simulink model "Headlight_dimmer"  (R2016a)
settings: Solver=VariableStepAuto  StartTime=0.0  StopTime=10.0  RelTol=1e-3
model workspace (MAT data in the model file):
  en = 0
  val = 0
  val1 = 0
values from neighbouring files (symbols this model uses):
  A = 1    [R_calculation_variables.mat]
  a = 0.7    [R_calculation_variables.mat]
libraries: simulink x3
settings Model: Creator=Admin  LastModifiedBy=Admin
settings DataIOCC: ExternalInput=[t, E]

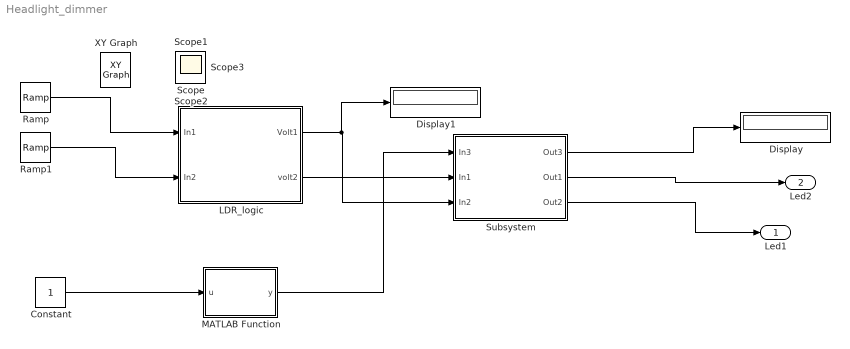
== system Headlight_dimmer ==
  Constant : Constant
  Display : Display
  Display1 : Display
  "LDR_logic " : Subsystem
  MATLAB Function : MATLAB Function  TreatAsAtomicUnit=on
  Ramp : simulink/Sources/Ramp  slope=0.5  start=0  X0=0
  Ramp1 : simulink/Sources/Ramp  slope=0.5  start=0  X0=0
  Subsystem : Subsystem
  Led1 : Outport
  Led2 : Outport  Port=2
  Scope{,1..3} (4 alike) : Scope
  XY Graph : simulink/Sinks/XY Graph  IOType=viewer  xmin=-1  xmax=1  ymin=-1  ymax=1  st=-1
  wires:
  Constant/1 -> MATLAB Function/1(u)
  Ramp/1 -> "LDR_logic "/1(In1)
  Ramp1/1 -> "LDR_logic "/2(In2)
  MATLAB Function/1(y) -> Subsystem/1(In3)
  "LDR_logic "/1(Volt1) -> Display1/1, Subsystem/3(In2)
  "LDR_logic "/2(volt2) -> Subsystem/2(In1)
  Subsystem/1(Out3) -> Display/1
  Subsystem/2(Out1) -> Led2/1
  Subsystem/3(Out2) -> Led1/1

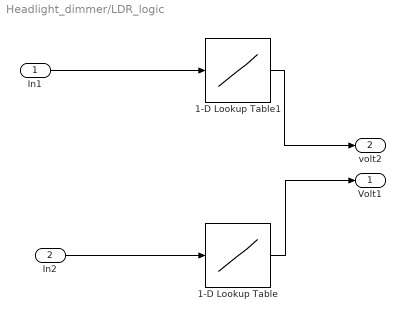
== system Headlight_dimmer/LDR_logic  ==
  In1 : Inport
  In2 : Inport  Port=2
  1-D Lookup Table : Lookup_n-D  NumberOfTableDimensions=1  BreakpointsForDimension1=A.*E.^a  Table=A.*E.^a  InternalRulePriority=Speed  RndMeth=Simplest  InputSameDT=on
  1-D Lookup Table1 : Lookup_n-D  NumberOfTableDimensions=1  BreakpointsForDimension1=A.*E.^a  Table=A.*E.^a  InternalRulePriority=Speed  RndMeth=Simplest  InputSameDT=on
  Volt1 : Outport
  volt2 : Outport  Port=2
  wires:
  1-D Lookup Table1/1 -> volt2/1
  1-D Lookup Table/1 -> Volt1/1
  In1/1 -> 1-D Lookup Table1/1
  In2/1 -> 1-D Lookup Table/1

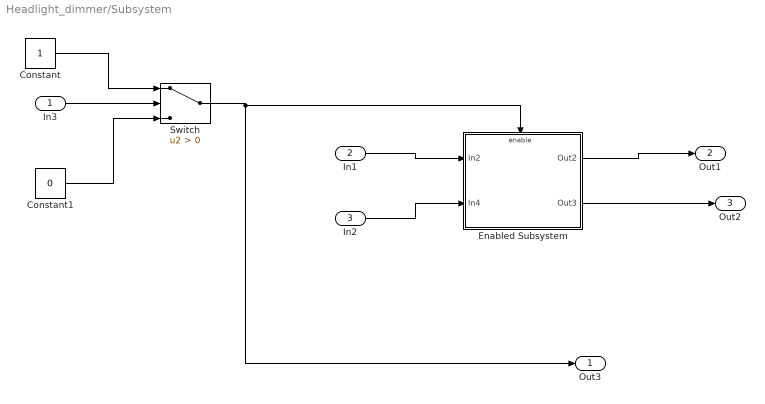
== system Headlight_dimmer/Subsystem ==
  In3 : Inport
  In1 : Inport  Port=2
  In2 : Inport  Port=3
  Constant : Constant
  Constant1 : Constant  Value=0
  Enabled Subsystem : Subsystem  TreatAsAtomicUnit=on
  Switch : Switch  Criteria=u2 > Threshold
  Out3 : Outport
  Out1 : Outport  Port=2
  Out2 : Outport  Port=3
  wires:
  In3/1 -> Switch/2
  Constant/1 -> Switch/1
  Constant1/1 -> Switch/3
  Switch/1 -> Enabled Subsystem/Enable, Out3/1
  Enabled Subsystem/2(Out3) -> Out2/1
  Enabled Subsystem/1(Out2) -> Out1/1
  In1/1 -> Enabled Subsystem/1(In2)
  In2/1 -> Enabled Subsystem/2(In4)

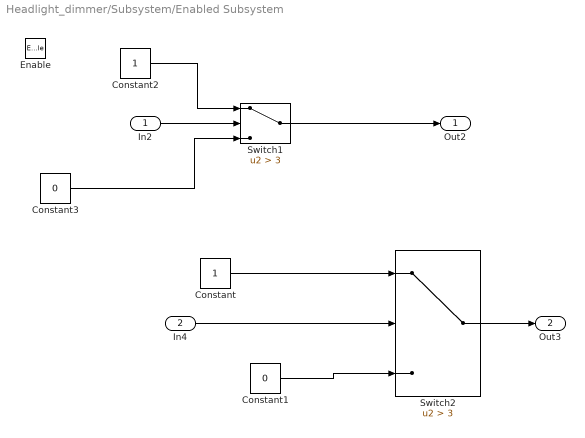
== system Headlight_dimmer/Subsystem/Enabled Subsystem ==
  In2 : Inport
  In4 : Inport  Port=2
  Enable : EnablePort
  Constant : Constant
  Constant1 : Constant  Value=0
  Constant2 : Constant
  Constant3 : Constant  Value=0
  Switch1 : Switch  Criteria=u2 > Threshold  Threshold=3
  Switch2 : Switch  Criteria=u2 > Threshold  Threshold=3
  Out2 : Outport
  Out3 : Outport  Port=2
  wires:
  Constant/1 -> Switch2/1
  Constant1/1 -> Switch2/3
  Switch2/1 -> Out3/1
  Switch1/1 -> Out2/1
  In2/1 -> Switch1/2
  In4/1 -> Switch2/2
  Constant2/1 -> Switch1/1
  Constant3/1 -> Switch1/3

== matlab function Headlight_dimmer/MATLAB Function ==
  data: u input; y output
function y = fcn(u)
%#codegen
   if u==1
       y=1;
   else
       y=0;
   end
end
